simulink model "Park_Transform"  (R2014b)
settings: Solver=ode45  StartTime=0.0  StopTime=10.0  RelTol=1e-3
settings Model: Creator=Eduardo Montilva  LastModifiedBy=Eduardo Montilva

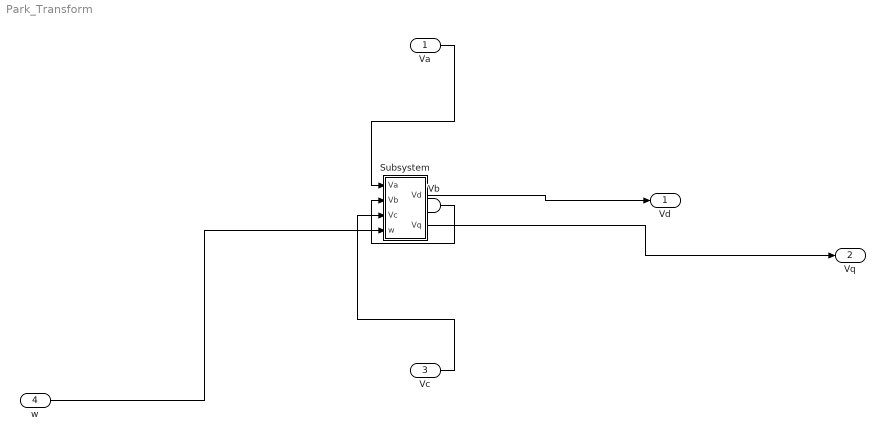
== system Park_Transform ==
  Va : Inport
  Vb : Inport  Port=2
  Vc : Inport  Port=3
  w : Inport  Port=4
  Subsystem : Subsystem
  Vd : Outport
  Vq : Outport  Port=2
  wires:
  Va/1 -> Subsystem/1(Va)
  Vb/1 -> Subsystem/2(Vb)
  Vc/1 -> Subsystem/3(Vc)
  w/1 -> Subsystem/4(w)
  Subsystem/1(Vd) -> Vd/1
  Subsystem/2(Vq) -> Vq/1

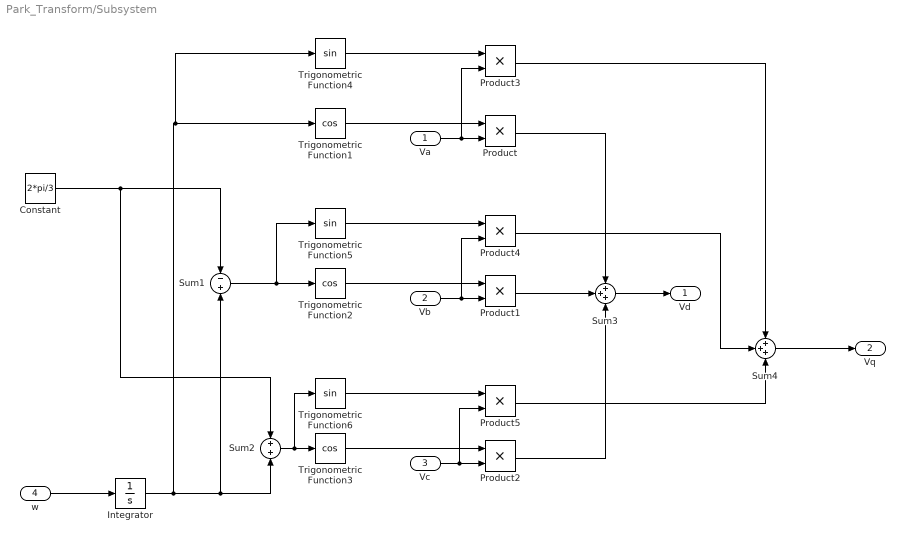
== system Park_Transform/Subsystem ==
  Va : Inport
  Vb : Inport  Port=2
  Vc : Inport  Port=3
  w : Inport  Port=4
  Constant : Constant  Value=2*pi/3
  Integrator : Integrator
  Product{,1..5} (6 alike) : Product
  Sum1 : Sum  Inputs=-+
  Sum2 : Sum
  Sum3 : Sum  Inputs=+++
  Sum4 : Sum  Inputs=+++
  Trigonometric Function1 : Trigonometry  Operator=cos
  Trigonometric Function2 : Trigonometry  Operator=cos
  Trigonometric Function3 : Trigonometry  Operator=cos
  Trigonometric Function4 : Trigonometry
  Trigonometric Function5 : Trigonometry
  Trigonometric Function6 : Trigonometry
  Vd : Outport
  Vq : Outport  Port=2
  wires:
  Trigonometric Function5/1 -> Product4/1
  Product5/1 -> Sum4/3
  Sum4/1 -> Vq/1
  Product1/1 -> Sum3/2
  Trigonometric Function2/1 -> Product1/1
  Trigonometric Function3/1 -> Product2/1
  Product/1 -> Sum3/1
  Vb/1 -> Product4/2, Product1/2
  Va/1 -> Product3/2, Product/2
  Product2/1 -> Sum3/3
  Vc/1 -> Product5/2, Product2/2
  Sum2/1 -> Trigonometric Function6/1, Trigonometric Function3/1
  Sum1/1 -> Trigonometric Function5/1, Trigonometric Function2/1
  Trigonometric Function1/1 -> Product/1
  Constant/1 -> Sum1/1, Sum2/1
  Sum3/1 -> Vd/1
  Trigonometric Function4/1 -> Product3/1
  Trigonometric Function6/1 -> Product5/1
  Product3/1 -> Sum4/1
  Product4/1 -> Sum4/2
  Integrator/1 -> Trigonometric Function4/1, Trigonometric Function1/1, Sum1/2, Sum2/2
  w/1 -> Integrator/1
